simulink model "uklad"  (R2021b)
settings: Solver=VariableStepAuto  StartTime=0.0  StopTime=10  RelTol=1e-3
undefined symbols (not defined in the file): b, c, d, x0
settings Model: Creator=Legion  LastModifiedBy=Legion

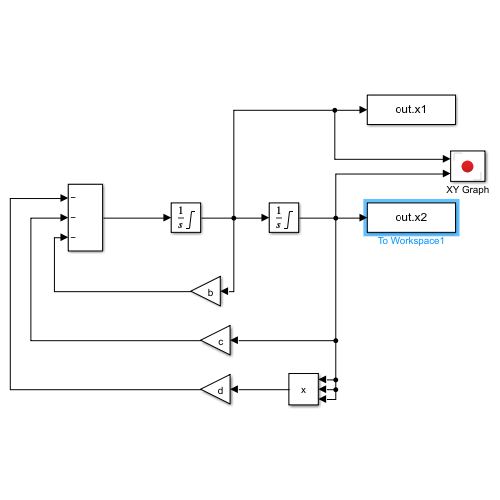
[thumbnail: Simulink's stored preview of the top-level diagram]
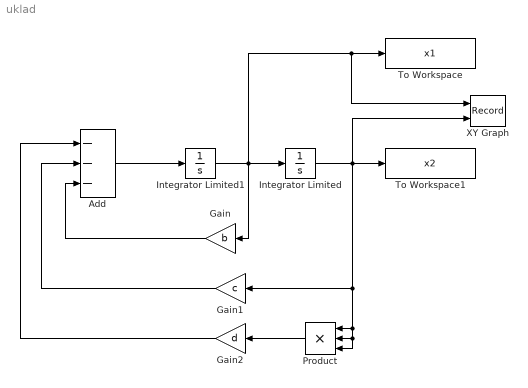
== system uklad ==
  Add : Sum  Inputs=---
  Gain : Gain  Gain=b
  Gain1 : Gain  Gain=c
  Gain2 : Gain  Gain=d
  Integrator Limited : Integrator  InitialCondition=x0(1)  LimitOutput=on  UpperSaturationLimit=2  LowerSaturationLimit=-2
  Integrator Limited1 : Integrator  InitialCondition=x0(2)  LimitOutput=on  UpperSaturationLimit=2  LowerSaturationLimit=-2
  Product : Product  Inputs=3
  To Workspace : ToWorkspace  VariableName=x1  SampleTime=-1
  To Workspace1 : ToWorkspace  VariableName=x2  SampleTime=-1
  XY Graph : Record  FileSettingsInternal="{\"entries\":[{\"content\":{\"excelSettings\":{\"content\":{},\"type\":\"Streamout.ExcelSettings\"}},\"type\":\"Streamout.FileSettingStorage\",\"uuid\":\"19108948-40a7-43bf-af90-d28d5dfe90f6\"}],\"packageUris\":[\"http://schema.mathworks.com/mf0/streamout_blocks/R2020a\"],\"version\":\"1.0\"}"  Layout=[1 1]  SignalsInternal="{\"entries\":[{\"content\":{\"signals\":[{\"content\":{\"blockPath\":[\"uklad/XY Graph\"],\"channel\":[],\"dimensions\":[1],\"domain\":\"uklad/XY Graph\",\"lineColor\":\"#a2142f\",\"plots\":[1],\"port\":1,\"sid\":[\"\"],\"signalID\":267,\"signalName\":\"Integrator\\nLimited1\"},\"type\":\"RecordBlkView.Signal\",\"uuid\":\"cd86a725-f064-4ede-a419-367942fe806c\"},{\"content\":{\"blockPath\":[\"uklad/XY Graph\"],\"channel\":[],\"dimensions\":[1],\"domain\":\"uklad/XY Graph\",\"lineColor\":\"#139fff\",\"plots\":[1],\"port\":2,\"sid\":[\"\"],\"signalID\":271,\"signalName\":\"Integrator\\nLimited\"},\"type\":\"RecordBlkView.Signal\",\"uuid\":\"cf94d3ce-4e13-4c9e-9180-dcae4a203538\"}]},\"type\":\"RecordBlkView.InputSignals\",\"uuid\":\"c29cc507-7b40-4165-89f6-e65ea39089ef\"}],\"packageUris\":[\"http://schema.mathworks.com/mf0/streamout_blocks/R2020a\"],\"version\":\"1.0\"}"  VisualizationBindings="{\"xyplotplugin\":{\"info\":[{\"series\":[{\"bindingParametersList\":[{\"parameter\":\"X-Axis\",\"signalID\":267,\"signalName\":\"Integrator\\nLimited1\"},{\"parameter\":\"Y-Axis\",\"signalID\":271,\"signalName\":\"Integrator\\nLimited\"}],\"seriesID\":50268}],\"subplotID\":1}]}}"  CompatibilityTag=XY
  wires:
  Add/1 -> Integrator Limited1/1
  Integrator Limited1/1 -> To Workspace/1, XY Graph/1, Gain/1, Integrator Limited/1
  Gain/1 -> Add/3
  Gain1/1 -> Add/2
  Gain2/1 -> Add/1
  Integrator Limited/1 -> To Workspace1/1, Product/3, Product/2, Product/1, Gain1/1, XY Graph/2
  Product/1 -> Gain2/1
